simulink model "Blackbox_MachineOne"  (R2020b)
settings: Solver=FixedStepAuto  StartTime=0.0  StopTime=inf  RelTol=1e-3  EnableMultiTasking=on
libraries: arduinolib x3
settings Model: SILPILModeSetting=veronly  ExtModeTrigDuration=2  Creator=nikhi  LastModifiedBy=nikhi
settings OptimizationCC: EnhancedBackFolding=on  PassReuseOutputArgsAs=Individual arguments  ZeroExternalMemoryAtStartup=off  ZeroInternalMemoryAtStartup=off  MaxStackSize=64  OptimizeBlockOrder=speed  DifferentSizesBufferReuse=on  OptimizationCustomize=off  EfficientTunableParamExpr=on
settings DebuggingCC: ParameterTunabilityLossMsg=error
settings HardwareCC: ProdBitPerInt=16  ProdBitPerPointer=16  ProdBitPerSizeT=16  ProdBitPerPtrDiffT=16  ProdLargestAtomicFloat=None  ProdWordSize=8  ProdHWDeviceType=Atmel->AVR  UseEmbeddedCoderFeatures=off  UseSimulinkCoderFeatures=off
settings SFSimCC: MATLABDynamicMemAlloc=off
settings RTWCC: Description=Embedded Coder  SystemTargetFile=ert.tlc  HardwareBoard=Arduino Uno  TemplateMakefile=ert_default_tmf  Toolchain=Arduino AVR  BuildConfiguration=Faster Runs
settings CodeAppCC: ForceParamTrailComments=on  IgnoreCustomStorageClasses=off  OperatorAnnotations=on  SimulinkDataObjDesc=on  SFDataObjDesc=on  InsertBlockDesc=on
settings ERTTargetCC: SupportContinuousTime=on  SupportNonInlinedSFcns=on  SupportVariableSizeSignals=on  ExtModeStaticAllocSize=250

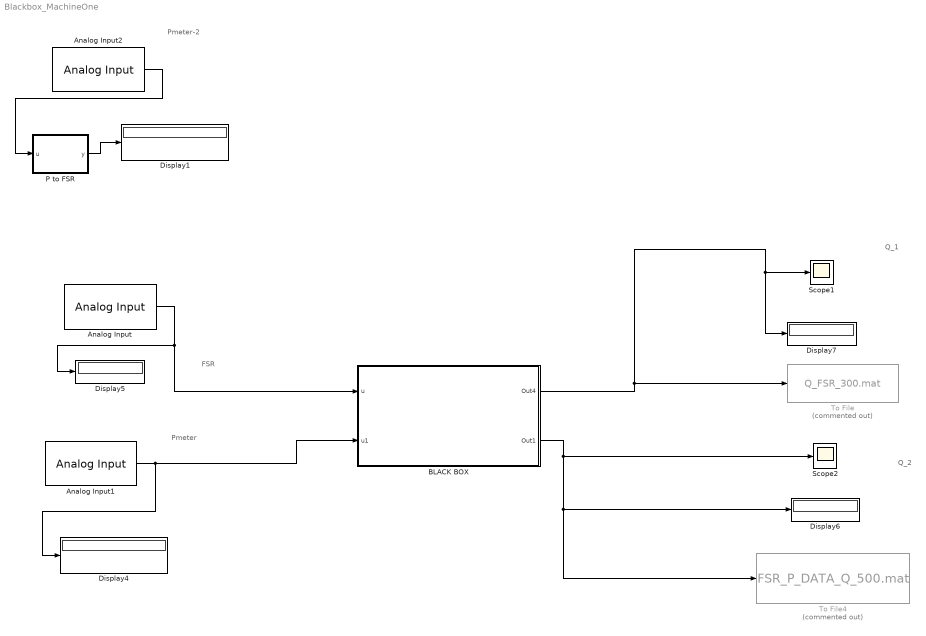
== system Blackbox_MachineOne ==
  note: Q_1
  note: Q_2
  note: FSR
  note: Pmeter
  note: Pmeter-2
  Analog Input : arduinolib/Analog Input  pinNumber=0  ReadResultsOnly=off  ConversionTriggerSource=Software  ExternalTriggerType=uint32( 0 )  OutputDataType=uint16  EnableConversionCompleteNotify=off  EnableOuputStatus=off  SampleTime=1  blockPlatform=arduino
  Analog Input1 : arduinolib/Analog Input  pinNumber=1  ReadResultsOnly=off  ConversionTriggerSource=Software  ExternalTriggerType=uint32( 0 )  OutputDataType=uint16  EnableConversionCompleteNotify=off  EnableOuputStatus=off  SampleTime=1  blockPlatform=arduino
  Analog Input2 : arduinolib/Analog Input  pinNumber=2  ReadResultsOnly=off  ConversionTriggerSource=Software  ExternalTriggerType=uint32( 0 )  OutputDataType=uint16  EnableConversionCompleteNotify=off  EnableOuputStatus=off  SampleTime=1  blockPlatform=arduino
  BLACK BOX : Subsystem
      mask Display: image('1.jfif'); % Use "Edit Image" on toolstrip to change.
  Display{1,4..7} (5 alike) : Display
  P to FSR : MATLAB Function  TreatAsAtomicUnit=on
  Scope1 : Scope
  Scope2 : Scope
  To File : ToFile  Commented=on  Filename=Q_FSR_300.mat  MatrixName=Q_FSR_300  SampleTime=1
      settings: Decimation=2
  To File4 : ToFile  Commented=on  Filename=FSR_P_DATA_Q_500.mat  MatrixName=FSR_P_DATA_Q_500  SampleTime=1
      settings: Decimation=2
  wires:
  Analog Input1/1 -> Display4/1, BLACK BOX/2(u1)
  Analog Input/1 -> BLACK BOX/1(u), Display5/1
  BLACK BOX/1(Out4) -> Display7/1, Scope1/1, To File/1
  BLACK BOX/2(Out1) -> To File4/1, Display6/1, Scope2/1
  Analog Input2/1 -> P to FSR/1(u)
  P to FSR/1(y) -> Display1/1

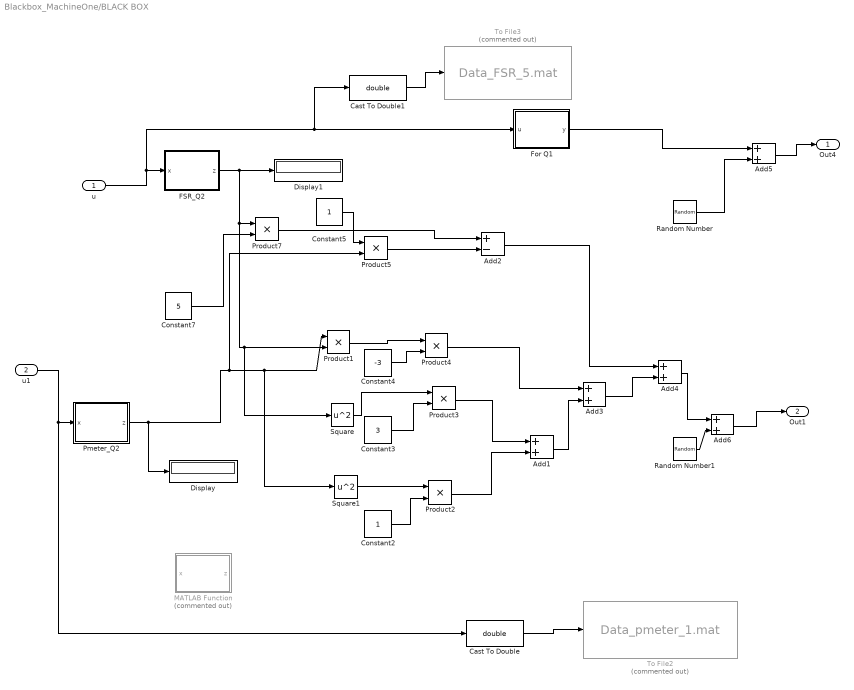
== system Blackbox_MachineOne/BLACK BOX ==
  u : Inport
  u1 : Inport  Port=2
  Add{1,3..6} (5 alike) : Sum
  Add2 : Sum  Inputs=+-
  Cast To Double : DataTypeConversion  OutDataTypeStr=double
  Cast To Double1 : DataTypeConversion  OutDataTypeStr=double
  Constant2 : Constant
  Constant3 : Constant  Value=3
  Constant4 : Constant  Value=-3
  Constant5 : Constant
  Constant7 : Constant  Value=5
  Display : Display
  Display1 : Display
  FSR_Q2 : MATLAB Function  TreatAsAtomicUnit=on
  For Q1 : MATLAB Function  TreatAsAtomicUnit=on
  MATLAB Function : MATLAB Function  Commented=on  TreatAsAtomicUnit=on
  Pmeter_Q2 : MATLAB Function  TreatAsAtomicUnit=on
  Product{1..5,7} (6 alike) : Product
  Random Number : RandomNumber  SampleTime=1  VectorParams1D=off
  Random Number1 : RandomNumber  SampleTime=1  VectorParams1D=off
  Square : Math  Operator=square  SaturateOnIntegerOverflow=on
  Square1 : Math  Operator=square  SaturateOnIntegerOverflow=on
  To File2 : ToFile  Commented=on  Filename=Data_pmeter_1.mat  MatrixName=Data_pmeter_1  SampleTime=1
      settings: Decimation=2
  To File3 : ToFile  Commented=on  Filename=Data_FSR_5.mat  MatrixName=Data_FSR_5  SampleTime=1
      settings: Decimation=2
  Out4 : Outport
  Out1 : Outport  Port=2
  wires:
  For Q1/1(y) -> Add5/1
  u1/1 -> Cast To Double/1, Pmeter_Q2/1(x)
  Square1/1 -> Product2/1
  Constant2/1 -> Product2/2
  Square/1 -> Product3/1
  Constant3/1 -> Product3/2
  Product1/1 -> Product4/1
  Constant4/1 -> Product4/2
  Constant5/1 -> Product5/1
  Product5/1 -> Add2/2
  Product3/1 -> Add1/1
  Product2/1 -> Add1/2
  Product4/1 -> Add3/1
  Add1/1 -> Add3/2
  Add3/1 -> Add4/2
  Add2/1 -> Add4/1
  Add4/1 -> Add6/1
  Constant7/1 -> Product7/2
  Random Number/1 -> Add5/2
  Add5/1 -> Out4/1
  Random Number1/1 -> Add6/2
  Add6/1 -> Out1/1
  u/1 -> Cast To Double1/1, For Q1/1(u), FSR_Q2/1(x)
  FSR_Q2/1(z) -> Product7/1, Square/1, Product1/2, Display1/1
  Pmeter_Q2/1(z) -> Display/1, Product5/2, Square1/1, Product1/1
  Cast To Double1/1 -> To File3/1
  Cast To Double/1 -> To File2/1
  Product7/1 -> Add2/1

== matlab function Blackbox_MachineOne/BLACK BOX/MATLAB Function ==
  data: x input; z output
function z = fcn(x)
% x - FSR; y - Pmeter
z = 0;
if x < 730
    z= 0;
elseif x >=730 && x<810
    z=100;
elseif x >810 && x < 850
    z= 200;
elseif x >850 && x < 885
    z=300;
elseif x >885 && x < 910
    z=400;
elseif x >910
    z=500;
end
z = z;

== matlab function Blackbox_MachineOne/BLACK BOX/Pmeter_Q2 ==
  data: x input; z output
function z = fcn(x)
% x - FSR; y - Pmeter
z = 0;
if x < 512
    z= ((double(x)*0.078) - 40);
elseif x ==512
    z=0;
elseif x >512
    z= double((x*0.078)- 40);
end
z = z;

== matlab function Blackbox_MachineOne/P to FSR ==
  data: u input; y output
function y = fcn(u)
x =u;
z= 0;
% x=-1:0.1:1;
if x < 690
    z = 100;
elseif x >=690 && x<740
    z = 200;
elseif x >=740 && x<780
    z= 300;
elseif x >780 && x < 800
    z= 400;
elseif x >800
    z= 500;
end
% plot(u,y)
% y = z - 6.325;
y = z;

== matlab function Blackbox_MachineOne/BLACK BOX/For Q1 ==
  data: u input; y output
function y = fcn(u)
x =u;
z= 0;
% x=-1:0.1:1;
if x < 740
    z=sqrt(double(4*22*x));
elseif x >=740 && x<780
    z=(sqrt(double(4*22*x))-(double(x*0.033)));
elseif x >780 && x < 800
    z=(sqrt(double(4*22*x))-(double(x*0.063)));
elseif x >800
    z=(sqrt(double(4*22*x))-(double(x*0.081)));
end
% plot(u,y)
% y = z - 6.325;
y = z;

== matlab function Blackbox_MachineOne/BLACK BOX/FSR_Q2 ==
  data: x input; z output
function z = fcn(x)
% x - FSR; y - Pmeter
z = 0;
if x < 500
    z= -25;
elseif x >=500 && x<680
    z=-12.5;
elseif x >=680 && x < 745
    z= 0;
elseif x >=745 && x<790
    z=12.5;
elseif x >=790
    z=25;
end
z = z;
